simulink model "chap7_10sim"  (Simulink 10.3)
settings: Solver=ode45  StartTime=0.0  StopTime=20  FixedStep=0.001  EnableMultiTasking=on
settings Model: Creator=shipe  LastModifiedBy=shipe
settings SolverCC: AlgebraicLoopSolver=Auto
settings DataIOCC: LimitDataPoints=on  SignalLoggingName=sigsOut
settings OptimizationCC: ExpressionDepthLimit=128  LifeSpan=auto
settings DebuggingCC: AlgebraicLoopMsg=none  SaveWithParameterizedLinksMsg=none  SignalResolutionControl=TryResolveAllWithWarning  MultiTaskDSMMsg=warning  MultiTaskCondExecSysMsg=none  FcnCallInpInsideContextMsg=error  StateNameClashWarn=none  SFUnexpectedBacktrackingDiag=error  SFNoUnconditionalDefaultTransitionDiag=error  SFExecutionAtInitializationDiag=warning  SFMachineParentedDataDiag=error  ArithmeticOperatorsInVariantConditions=error
settings HardwareCC: TargetUnknown=on
settings SFSimCC: SimUseLocalCustomCode=on  CustomCodeUndefinedFunction=FilterOut
settings RTWCC: RTWUseLocalCustomCode=on
settings CodeAppCC: StateflowObjectComments=off
settings GRTTargetCC: TargetLangStandard=C99 (ISO)
settings ConfigComp: CovExternalEMLEnable=on

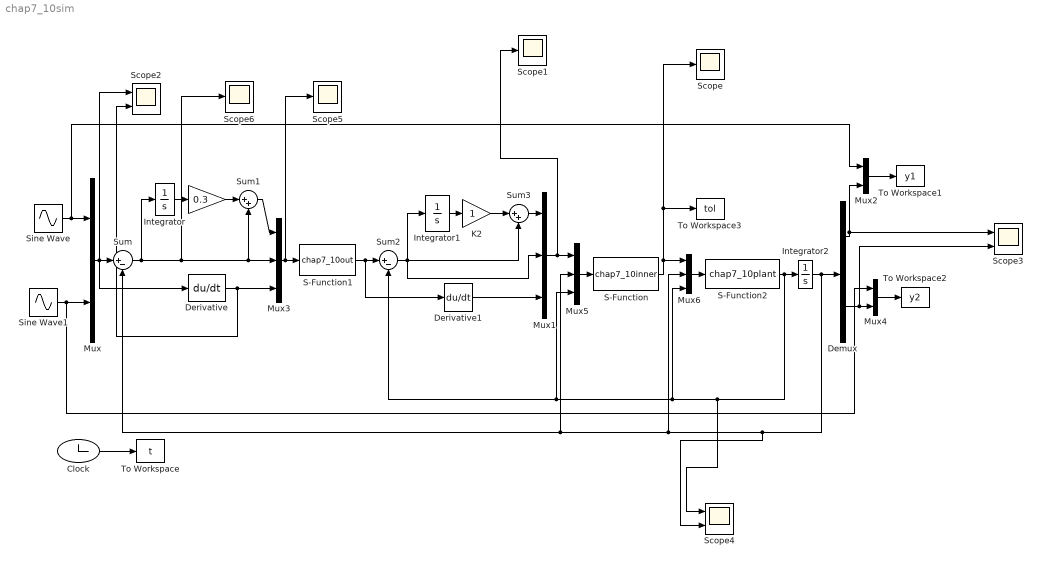
== system chap7_10sim ==
  " " : Gain  Gain=0.3  SaturateOnIntegerOverflow=on  OutDataTypeStr=Inherit: Same as input  ParamDataTypeStr=Inherit: Same as input
  Clock : Clock
  Demux : Demux  Outputs=2
      settings: DisplayOption=none
  Derivative : Derivative
  Derivative1 : Derivative
  Integrator : Integrator
  Integrator1 : Integrator
  Integrator2 : Integrator
  K2 : Gain  SaturateOnIntegerOverflow=on  OutDataTypeStr=Inherit: Same as input  ParamDataTypeStr=Inherit: Same as input
  Mux : Mux  Inputs=2
  Mux{1,3,5..6} (4 alike) : Mux  Inputs=3
  Mux2 : Mux  Inputs=2
  Mux4 : Mux  Inputs=2
  S-Function : S-Function  FunctionName=chap7_10inner  SFunctionDeploymentMode=off  EnableBusSupport=off
  S-Function1 : S-Function  FunctionName=chap7_10out  SFunctionDeploymentMode=off  EnableBusSupport=off
  S-Function2 : S-Function  FunctionName=chap7_10plant  SFunctionDeploymentMode=off  EnableBusSupport=off
  Scope{,1,5..6} (4 alike) : Scope
  Scope2 : Scope  NumInputPorts=2
  Scope3 : Scope  NumInputPorts=2
  Scope4 : Scope  NumInputPorts=2
  Sine Wave : Sin  Phase=pi/2  SampleTime=0
  Sine Wave1 : Sin  Phase=pi/2  SampleTime=0
  Sum : Sum  Inputs=|+-  SaturateOnIntegerOverflow=on
  Sum1 : Sum  Inputs=|++  SaturateOnIntegerOverflow=on
  Sum2 : Sum  Inputs=|+-  SaturateOnIntegerOverflow=on
  Sum3 : Sum  Inputs=|++  InputSameDT=on  SaturateOnIntegerOverflow=on  OutDataTypeStr=Inherit: Same as first input
  To Workspace : ToWorkspace  VariableName=t  SampleTime=-1
  To Workspace1 : ToWorkspace  VariableName=y1  SampleTime=-1
  To Workspace2 : ToWorkspace  VariableName=y2  SampleTime=-1
  To Workspace3 : ToWorkspace  VariableName=tol  SampleTime=-1
  wires:
  S-Function2/1 -> Integrator2/1, Scope4/1, Mux6/3, Mux5/3, Sum2/2
  Sine Wave/1 -> Mux/1, Mux2/1
  Integrator2/1 -> Demux/1, Scope4/2, Sum/2, Mux5/2, Mux6/2
  Sum/1 -> Scope6/1, Sum1/2, Mux3/2, Integrator/1
  Integrator/1 -> " "/1
  " "/1 -> Sum1/1
  Derivative/1 -> Scope2/2, Mux3/3
  Mux3/1 -> Scope5/1, S-Function1/1
  S-Function1/1 -> Derivative1/1, Sum2/1
  Sum2/1 -> Integrator1/1, Sum3/2, Mux1/2
  Integrator1/1 -> K2/1
  K2/1 -> Sum3/1
  Sum3/1 -> Mux1/1
  Derivative1/1 -> Mux1/3
  Mux/1 -> Scope2/1, Sum/1, Derivative/1
  Sine Wave1/1 -> Mux4/1, Mux/2
  Demux/1 -> Mux2/2, Scope3/1
  Mux2/1 -> To Workspace1/1
  Mux4/1 -> To Workspace2/1
  Demux/2 -> Scope3/2, Mux4/2
  Mux5/1 -> S-Function/1
  Mux6/1 -> S-Function2/1
  S-Function/1 -> Mux6/1, Scope/1, To Workspace3/1
  Clock/1 -> To Workspace/1
  Mux1/1 -> Scope1/1, Mux5/1
  Sum1/1 -> Mux3/1
